simulink library "gtkWave"  (Simulink 7.1)
undefined symbols (not defined in the file or in its folder): gtkStartFcn
libraries: xbsIndex_r4 x4
settings Model: Creator=Glenn  LastModifiedBy=Glenn

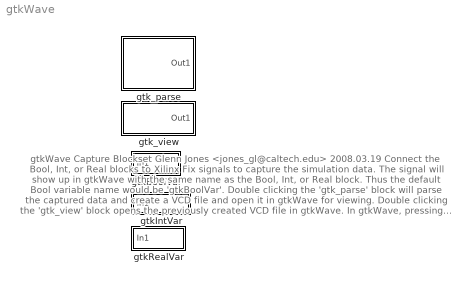
== system gtkWave ==
  note: gtkWave Capture Blockset
      | Glenn Jones <jones_gl@caltech.edu>
      | 2008.03.19
      |
      | Connect the Bool, Int, or Real blocks to Xilinx Fix signals to capture
      | the simulation data. The signal will show up in gtkWave with the same
      | name as the Bool, Int, or Real block. Thus the default Bool variable name
      | would be 'gtkBoolVar'.
      | Double clicking the 'gtk_parse' block will parse the captured data
      | and create a VCD file and open it in gtkWave for viewing.
      | Double clicking the 'gtk_view' block opens the previously created VCD
      | file in gtkWave.
      | In gtkWave, pressing 'File/Write Save File' or 'ctrl-S' will save the current
      | viewing settings. These settings will be reloaded automatically the next
      | time 'gtk_parse' or 'gtk_view' is run.
      |
      | Notes:
      | 1. You must not name any variables with names starting 'gtk_'
      | 2. By default, the signals in gtkWave are simply named after the block that
      | captured them. If you create a variable in the workspace called
      | 'full_path_gtk', the signals will be named with the full path heirarchy. This
      | aids clarity, but takes up plotting real estate.
  gtkBoolVar : Subsystem
      mask help: Capture a Boolean signal to view in gtkWave.
      mask init:
      | gtkBool_init
      mask Display: disp('gtkBool')
  gtkIntVar : Subsystem  mask{width=32}
      mask prompts: width "Bit Width"
      mask help:
      | Capture an Integer signal to view in gtkWave.
      | gtkWave does not support fixed point variables, so all integers will appear with binary point at 0.
      | The input signal to this block should be less than 50 bits wide, as it is represented in Matlab as a double.
      mask init:
      | gtkFix_init
      mask Display: disp(['gtkFix',num2str(width)])
  gtkRealVar : Subsystem
      mask help:
      | Capture a Real variable to view in gtkWave.
      | Input is a Xilinx Fix interpreted as a real number.
      mask init:
      | gtkReal_init
      mask Display: disp('gtkReal')
  gtk_parse : Subsystem  StartFcn=gtkStartFcn()  mask(gtk_parse){dummy=0}
      mask help: asdf
      settings: OpenFcn=gtk_parse()
      mask Display: fprintf('Double Click\nTo make and\nView VCD')
  gtk_view : Subsystem
      settings: OpenFcn=gtk_view()
      mask Type: gtk_view
      mask Description: asdf
      mask Display: disp('View VCD')

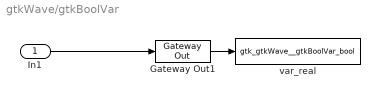
== system gtkWave/gtkBoolVar ==
  In1 : Inport  OutDataType=sfix(16)  OutScaling=2^0
  Gateway Out1 : xbsIndex_r4/Gateway Out  hdl_port=off  timing_constraint=None  locs_specified=off  LOCs={}  block_type=gatewayout
      settings: infoedit="Gateway out block.  Converts Xilinx fixed point inputs into ouputs of type Simulink integer, double, or fixed point.<P><P>Hardware notes:  In hardware these blocks become top level output ports or are discarded, depending on how they are configured."  xl_area=[0, 0, 0, 0, 0, 0, 0]  block_version=10.1.2
  var_real : ToWorkspace  VariableName=gtk_gtkWave__gtkBoolVar_bool  SampleTime=-1  SaveFormat=Structure With Time
  wires:
  Gateway Out1/1 -> var_real/1
  In1/1 -> Gateway Out1/1

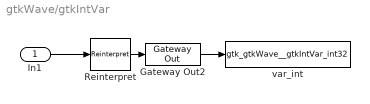
== system gtkWave/gtkIntVar ==
  In1 : Inport  OutDataType=sfix(16)  OutScaling=2^0
  Gateway Out2 : xbsIndex_r4/Gateway Out  hdl_port=off  timing_constraint=None  locs_specified=off  LOCs={}  block_type=gatewayout
      settings: infoedit="Gateway out block.  Converts Xilinx fixed point inputs into ouputs of type Simulink integer, double, or fixed point.<P><P>Hardware notes:  In hardware these blocks become top level output ports or are discarded, depending on how they are configured."  xl_area=[0, 0, 0, 0, 0, 0, 0]  block_version=10.1.2
  Reinterpret : xbsIndex_r4/Reinterpret  force_arith_type=on  arith_type=Unsigned  force_bin_pt=on  bin_pt=0  block_type=reinterpret
      settings: infoedit="Changes signal type without altering the binary representation.   You can changed the signal between signed and unsigned, and relocate the binary point.<P><P>Hardware notes: In hardware this block costs nothing.<P><P>Example:  Suppose the input is 6 bits wide, signed, with 2 fractional bits, and the output is forced to unsigned with 0 fractional bits.  Then an input of -2.0 (1110.00 in binary 2's complement) becomes an output of 56 (111000 in binary)."  block_version=10.1.2
  var_int : ToWorkspace  VariableName=gtk_gtkWave__gtkIntVar_int32  SampleTime=-1  SaveFormat=Structure With Time
  wires:
  Reinterpret/1 -> Gateway Out2/1
  Gateway Out2/1 -> var_int/1
  In1/1 -> Reinterpret/1

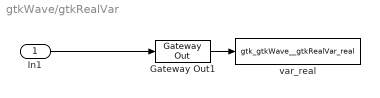
== system gtkWave/gtkRealVar ==
  In1 : Inport  OutDataType=sfix(16)  OutScaling=2^0
  Gateway Out1 : xbsIndex_r4/Gateway Out  hdl_port=off  timing_constraint=None  locs_specified=off  LOCs={}  block_type=gatewayout
      settings: infoedit="Gateway out block.  Converts Xilinx fixed point inputs into ouputs of type Simulink integer, double, or fixed point.<P><P>Hardware notes:  In hardware these blocks become top level output ports or are discarded, depending on how they are configured."  xl_area=[0, 0, 0, 0, 0, 0, 0]  block_version=10.1.2
  var_real : ToWorkspace  VariableName=gtk_gtkWave__gtkRealVar_real  SampleTime=-1  SaveFormat=Structure With Time
  wires:
  Gateway Out1/1 -> var_real/1
  In1/1 -> Gateway Out1/1

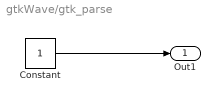
== system gtkWave/gtk_parse ==
  Constant : Constant  OutDataType=sfix(16)  OutScaling=2^0
  Out1 : Outport  OutDataType=sfix(16)  OutScaling=2^0
  wires:
  Constant/1 -> Out1/1

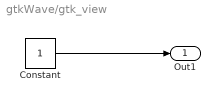
== system gtkWave/gtk_view ==
  Constant : Constant  OutDataType=sfix(16)  OutScaling=2^0
  Out1 : Outport  OutDataType=sfix(16)  OutScaling=2^0
  wires:
  Constant/1 -> Out1/1
